simulink subsystem "DM_SystemDiagnostics"  (R2019b)
settings: Solver=VariableStepAuto  StartTime=0.0  StopTime=10.0  RelTol=1e-3
settings Model: Creator=Nick  LastModifiedBy=Nick

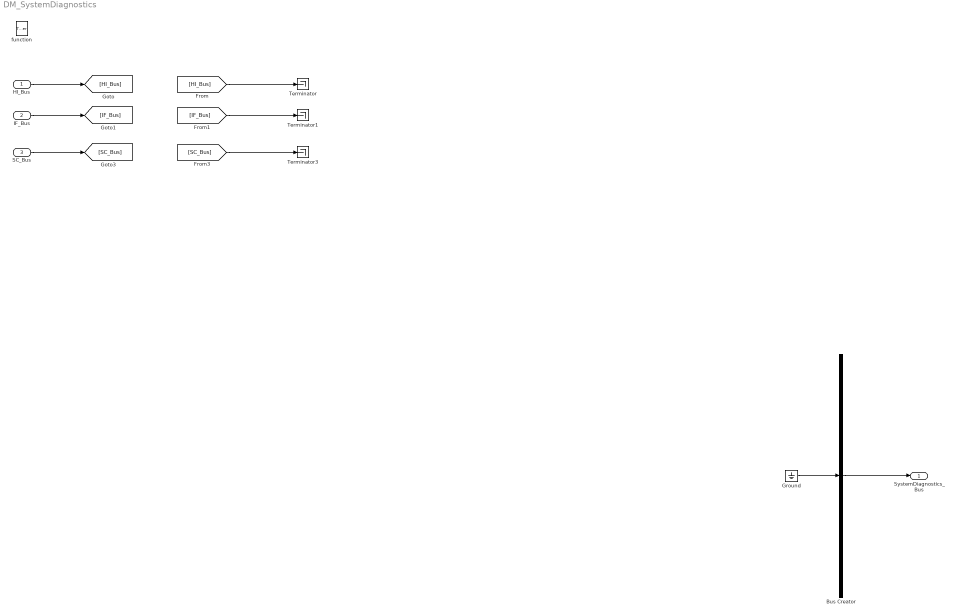
== system DM_SystemDiagnostics ==
  HI_Bus : Inport
  IF_Bus : Inport  Port=2
  SC_Bus : Inport  Port=3
  function : TriggerPort  TriggerType=function-call  VariantControl=Variant
  Bus Creator : BusCreator  Inputs=1
  Ground : Ground
  Terminator : Terminator
  Terminator1 : Terminator
  Terminator3 : Terminator
  SystemDiagnostics_Bus : Outport
  wires:
  [IF_Bus] -> Terminator1/1
  [HI_Bus] -> Terminator/1
  IF_Bus/1 -> [IF_Bus]
  HI_Bus/1 -> [HI_Bus]
  [SC_Bus] -> Terminator3/1
  SC_Bus/1 -> [SC_Bus]
  Bus Creator/1 -> SystemDiagnostics_Bus/1
  Ground/1 -> Bus Creator/1
